simulink model "motor_p"  (Simulink 3.00)
libraries: mathlib x13, genlib x3, reglib x2, arclib x2

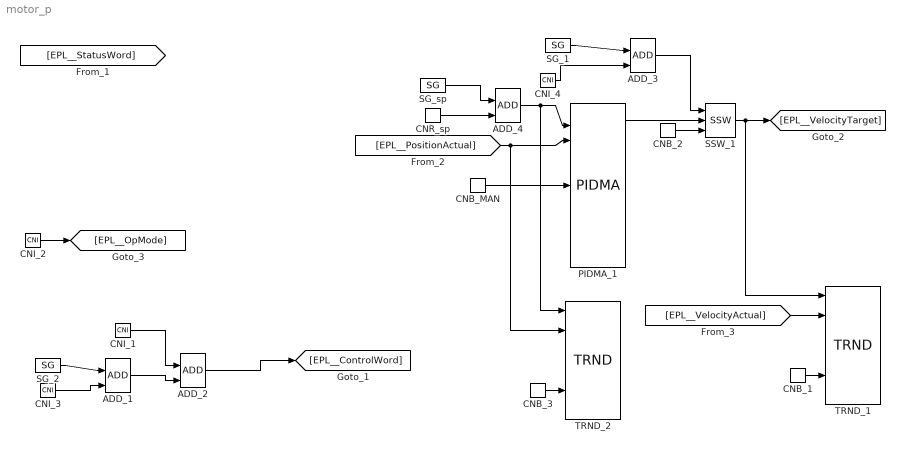
== system motor_p ==
  ADD_{1..4} (4 alike) : mathlib/ADD
  CNB_1 : mathlib/CNB  YCN=on
  CNB_2 : mathlib/CNB  YCN=on
  CNB_3 : mathlib/CNB  YCN=on
  CNB_MAN : mathlib/CNB  YCN=on
  CNI_1 : mathlib/CNI  icn=15
  CNI_2 : mathlib/CNI  icn=3
  CNI_3 : mathlib/CNI  icn=64
  CNI_4 : mathlib/CNI  icn=0
  CNR_sp : mathlib/CNR  ycn=1
  PIDMA_1 : reglib/PIDMA  irtype=4: P  RACT=off  k=0.01  ti=4  td=1  nd=10  b=1  c=0  tt=1  hilim=500  lolim=-500  dz=0  icotype=1: Analog  ittype=6: PI  iainf=1: Static process  DGC=on  tdg=60  tn=5  amp=0.5  dy=0.1  ispeed=2: Normal (middle fast) CL  ipid=1: Parallel form
  SG_1 : genlib/SG  isig=2: SQUARE  amp=0  freq=0.05  phase=0  ifrunit=1: Hz  iphunit=1: degree
  SG_2 : genlib/SG  isig=2: SQUARE  amp=64  freq=0.1  phase=0  ifrunit=1: Hz  iphunit=1: degree
  SG_sp : genlib/SG  isig=2: SQUARE  amp=0  freq=0.05  phase=0  ifrunit=1: Hz  iphunit=1: degree
  SSW_1 : reglib/SSW
  TRND_1 : arclib/TRND  n=4  l=1000  btype=8: Double  ptype1=1: Store  ptype2=1: Store  ptype3=1: Store  ptype4=1: Store  pfac=1  afac=0  arc=0  id=1  Title=Trend Title
  TRND_2 : arclib/TRND  n=4  l=1000  btype=8: Double  ptype1=1: Store  ptype2=1: Store  ptype3=1: Store  ptype4=1: Store  pfac=1  afac=0  id=2  Title=Trend Title
  wires:
  ADD_1/1 -> ADD_2/2
  ADD_2/1 -> [EPL__ControlWord]
  ADD_3/1 -> SSW_1/1
  ADD_4/1 -> PIDMA_1/2, TRND_2/1
  CNB_1/1 -> TRND_1/5
  CNB_2/1 -> SSW_1/3
  CNB_3/1 -> TRND_2/5
  CNB_MAN/1 -> PIDMA_1/6
  CNI_1/1 -> ADD_2/1
  CNI_2/1 -> [EPL__OpMode]
  CNI_3/1 -> ADD_1/2
  CNI_4/1 -> ADD_3/2
  CNR_sp/1 -> ADD_4/2
  [EPL__PositionActual] -> PIDMA_1/3, TRND_2/2
  [EPL__VelocityActual] -> TRND_1/2
  PIDMA_1/1 -> SSW_1/2
  SG_1/1 -> ADD_3/1
  SG_2/1 -> ADD_1/1
  SG_sp/1 -> ADD_4/1
  SSW_1/1 -> [EPL__VelocityTarget], TRND_1/1
